simulink model "Messages8"  (R2020a)
settings: Solver=FixedStepDiscrete  StartTime=0.0  StopTime=5  FixedStep=1  RelTol=1e-3  EnableMultiTasking=on
undefined symbols (not defined in the file or in its folder): m, n
settings Model: Creator=The MathWorks, Inc.  LastModifiedBy=bzhan
settings DataIOCC: LimitDataPoints=on  SaveFormat=Array  ReturnWorkspaceOutputs=off
settings OptimizationCC: ExpressionDepthLimit=2147483647  LifeSpan=1  EfficientTunableParamExpr=on
settings DebuggingCC: UnderspecifiedInitializationDetection=Classic  MergeDetectMultiDrivingBlocksExec=none  SolverPrmCheckMsg=warning  AllowSymbolicDim=off  StateNameClashWarn=warning  SFUnexpectedBacktrackingDiag=warning  SFNoUnconditionalDefaultTransitionDiag=warning  SFExecutionAtInitializationDiag=none  ArithmeticOperatorsInVariantConditions=warning
settings HardwareCC: ProdBitPerPointer=32  ProdBitPerSizeT=32  ProdBitPerPtrDiffT=32  ProdLargestAtomicFloat=None  ProdIntDivRoundTo=Undefined  ProdEndianess=Unspecified  ProdWordSize=32  ProdHWDeviceType=32-bit Generic
settings ModelReferenceCC: PropagateSignalLabelsOutOfModel=off
settings SFSimCC: SimUseLocalCustomCode=off  MATLABDynamicMemAlloc=off  CustomCodeUndefinedFunction=UseInterfaceOnly
settings RTWCC: Description=Real-Time Workshop Embedded Coder  SystemTargetFile=ert.tlc  TemplateMakefile=ert_default_tmf  RTWUseLocalCustomCode=off
settings CodeAppCC: IgnoreCustomStorageClasses=off  CustomSymbolStrType=$N$R$M  StateflowObjectComments=on  InternalIdentifier=Classic
settings ERTTargetCC: MultiwordLength=2048  GenerateSampleERTMain=on  ERTCustomFileTemplate=example_file_process.tlc  ConvertIfToSwitch=off  SuppressUnreachableDefaultCases=off
settings ConfigComp: CovMetricSettings=dw  CovHtmlReporting=on  CovSaveCumulativeToWorkspaceVar=on  CovSaveSingleToWorkspaceVar=on  CovExternalEMLEnable=off  CovSFcnEnable=off

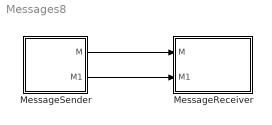
== system Messages8 ==
  MessageReceiver : Stateflow chart  TreatAsAtomicUnit=on
  MessageSender : Stateflow chart  TreatAsAtomicUnit=on
  wires:
  MessageSender/1(M) -> MessageReceiver/1(M)
  MessageSender/2(M1) -> MessageReceiver/2(M1)

== stateflow chart Messages8/MessageSender ==
  state A
    en:
    f("en_A");
    M.data=2;
    send(M);
    M1.data=3;
    send(M1);
  (default) -> A
  data: s function_input; M output double; M1 output
  function f(s):
    | function f(s)
    |   fprintf(s+"\n");

== stateflow chart Messages8/MessageReceiver ==
  settings: updateMethod=DISCRETE  sampleTime=1
  state A0
    en:f("en_A0");
  state A1
    en:f("en_A1");
  state A2
    en:f("en_A2");
  state A3
    en:f("en_A3");
  (default) -> A0
  A0 -> A1 : after(3,sec)
  A1 -> A2 : M[M.data==2]
  A2 -> A3 : M1[M1.data==3]
  data: s function_input; M input double; M1 input
  function f(s):
    | function f(s)
    |   fprintf(s+"\n");
